simulink model "TD2_NL_MODEL"  (Simulink 7.6)
settings: Solver=ode45  StartTime=0.0  StopTime=20  RelTol=1e-3
libraries: simulink x1, ADRC x1
settings Model: Creator=Administrator  LastModifiedBy=Administrator
settings DebuggingCC: SolverPrmCheckMsg=none

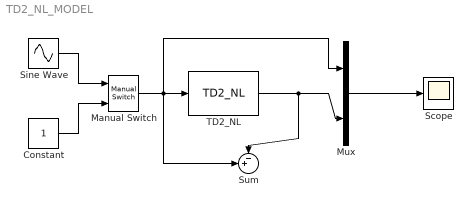
== system TD2_NL_MODEL ==
  Constant : Constant  SampleTime=0.01
  Manual Switch : simulink/Signal Routing/Manual Switch  SystemSampleTime=-1  sw=0  action=0  varsize=off
  Mux : Mux  Inputs=2
  Scope : Scope
      settings: TickLabels=on  TimeRange=20  YMin=-0.05  YMax=1.05  DataFormat=Array
  Sine Wave : Sin  Frequency=pi/2  SampleTime=0
  Sum : Sum  Inputs=-+|
  TD2_NL : ADRC/TD/TD2_NL/TD2_NL  r=20  h=0.01  h0=0
  wires:
  Manual Switch/1 -> Mux/1, Sum/2, TD2_NL/1
  Mux/1 -> Scope/1
  TD2_NL/1 -> Mux/2, Sum/1
  Sine Wave/1 -> Manual Switch/1
  Constant/1 -> Manual Switch/2
